simulink model "RflysimIndoorController_r2018b_N12_V9"  (R2018b)
settings: Solver=ode4  StartTime=0.0  StopTime=inf  FixedStep=ts  MaxStep=0.6  RelTol=1e-3
values from neighbouring files (symbols this model uses):
  l_v = 5    [RflyMain.m]    (also in RflyMain_N12_V6.m; RflyMain_N6_V3.m; RflyMain_N6_V4.m; RflyMain_V2.m)
  p_target = [200,10]    [RflyMain.m]    (also in RflyMain_N12_V6.m; RflyMain_N6_V3.m; RflyMain_N6_V4.m; RflyMain_V2.m)
  ra = 0.6    [RflyMain.m]    (also in RflyMain_N12_V6.m; RflyMain_N6_V3.m; RflyMain_N6_V4.m; RflyMain_V2.m)
  rs = 0.25    [RflyMain.m]    (also in RflyMain_N12_V6.m; RflyMain_N6_V3.m; RflyMain_N6_V4.m; RflyMain_V2.m)
  rt_a = 1.5    [RflyMain_N12_V6.m]
  rt_s = 0.25    [RflyMain_N12_V6.m]
  ts = [0 0]    [QuadModel2D.m]    (also in RflyMain.m = 0.01; RflyMain_N12_V6.m = 0.05; RflyMain_N6_V3.m = 0.05; RflyMain_N6_V4.m = 0.05)
  v_max = 2    [RflyMain.m]    (also in RflyMain_N12_V6.m = 3; RflyMain_N6_V3.m = 3; RflyMain_N6_V4.m = 3; RflyMain_V2.m = 3)
undefined symbols (not defined in the file or in its folder): Twist
libraries: robotlib x96, aerolibanimutils x1
(part 1 of 2)
settings Model: Creator=51078  LastModifiedBy=51078
settings OptimizationCC: EnhancedBackFolding=on  PassReuseOutputArgsAs=Individual arguments  ZeroExternalMemoryAtStartup=off  ZeroInternalMemoryAtStartup=off  MaxStackSize=64  OptimizeBlockOrder=speed  DifferentSizesBufferReuse=on  OptimizationCustomize=off
settings DebuggingCC: RTPrefix=warning  ParameterTunabilityLossMsg=error
settings HardwareCC: ProdBitPerPointer=32  ProdBitPerSizeT=32  ProdBitPerPtrDiffT=32  ProdLargestAtomicFloat=None  ProdIntDivRoundTo=Undefined  ProdEndianess=Unspecified  ProdWordSize=32  ProdHWDeviceType=Generic->Unspecified (assume 32-bit Generic)
settings SFSimCC: SimUseLocalCustomCode=off  MATLABDynamicMemAlloc=off
settings RTWCC: SystemTargetFile=ert.tlc  HardwareBoard=Robot Operating System (ROS)  TLCOptions="-aInlineSetEventsForThisBaseRateFcn=TLC_FALSE -aSuppressMultiTaskScheduler=TLC_FALSE  -aRateBasedStepFcn=0"  TemplateMakefile=ert_default_tmf  RTWUseLocalCustomCode=off  Toolchain=Catkin  TargetLang=C++
settings CodeAppCC: ForceParamTrailComments=on  IgnoreCustomStorageClasses=off  OperatorAnnotations=on  SimulinkDataObjDesc=on  SFDataObjDesc=on  InsertBlockDesc=on
settings ERTTargetCC: SupportVariableSizeSignals=on

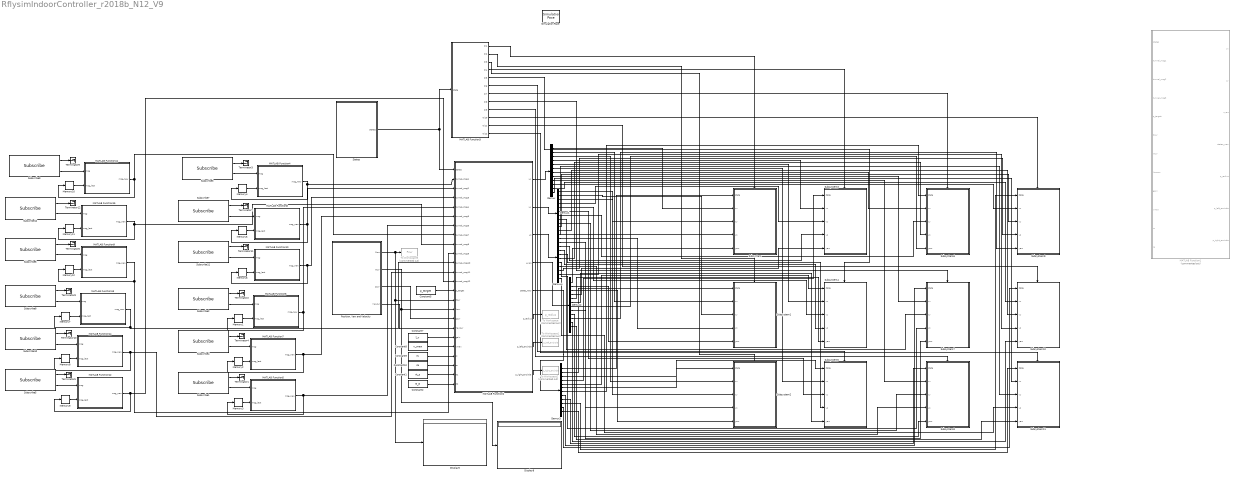
== system RflysimIndoorController_r2018b_N12_V9 ==
  Constant1 : Constant  Value=rt_s
  Constant10 : Constant  Value=ra
  Constant2 : Constant  Value=rt_a
  Constant5 : Constant  Value=p_target
  Constant7 : Constant  Value=l_v
  Constant8 : Constant  Value=v_max
  Constant9 : Constant  Value=rs
  Demux{,1..4} (5 alike) : Demux  Outputs=12
  Display6 : Display
  Display8 : Display
  MATLAB Function1 : MATLAB Function  Commented=on  TreatAsAtomicUnit=on
  MATLAB Function10 : MATLAB Function  TreatAsAtomicUnit=on
  MATLAB Function11 : MATLAB Function  TreatAsAtomicUnit=on
  MATLAB Function12 : MATLAB Function  TreatAsAtomicUnit=on
  MATLAB Function13 : MATLAB Function  TreatAsAtomicUnit=on
  MATLAB Function14 : MATLAB Function  TreatAsAtomicUnit=on
  MATLAB Function15 : MATLAB Function  TreatAsAtomicUnit=on
  MATLAB Function2 : MATLAB Function  TreatAsAtomicUnit=on
  MATLAB Function3 : MATLAB Function  TreatAsAtomicUnit=on
  MATLAB Function4 : MATLAB Function  TreatAsAtomicUnit=on
  MATLAB Function5 : MATLAB Function  TreatAsAtomicUnit=on
  MATLAB Function6 : MATLAB Function  TreatAsAtomicUnit=on
  MATLAB Function7 : MATLAB Function  TreatAsAtomicUnit=on
  MATLAB Function8 : MATLAB Function  TreatAsAtomicUnit=on
  MATLAB Function9 : MATLAB Function  TreatAsAtomicUnit=on
  Memory{1..12} (12 alike) : Memory
  "Position, Yaw and Velocity" : Subsystem
  Simulation Pace : aerolibanimutils/Simulation Pace  SimulationPace=1  SleepMode=MATLAB Thread  OutputPaceError=off  SampleTime=ts
  States : Subsystem
  Subscribe1 : robotlib/Subscribe  topicSource=Specify your own  topic=/drone_6/decision_info  messageType=swarm_msgs/Pipeline  sampleTime=-1  messageQueueLength=1
  Subscribe10 : robotlib/Subscribe  topicSource=Specify your own  topic=/drone_11/decision_info  messageType=swarm_msgs/Pipeline  sampleTime=-1  messageQueueLength=1
  Subscribe11 : robotlib/Subscribe  topicSource=Select from ROS network  topic=/drone_3/decision_info  messageType=swarm_msgs/Pipeline  sampleTime=-1  messageQueueLength=1
  Subscribe12 : robotlib/Subscribe  topicSource=Specify your own  topic=/drone_8/decision_info  messageType=swarm_msgs/Pipeline  sampleTime=-1  messageQueueLength=1
  Subscribe2 : robotlib/Subscribe  topicSource=Specify your own  topic=/drone_4/decision_info  messageType=swarm_msgs/Pipeline  sampleTime=-1  messageQueueLength=1
  Subscribe3 : robotlib/Subscribe  topicSource=Select from ROS network  topic=/drone_1/decision_info  messageType=swarm_msgs/Pipeline  sampleTime=-1  messageQueueLength=1
  Subscribe4 : robotlib/Subscribe  topicSource=Specify your own  topic=/drone_5/decision_info  messageType=swarm_msgs/Pipeline  sampleTime=-1  messageQueueLength=1
  Subscribe5 : robotlib/Subscribe  topicSource=Specify your own  topic=/drone_12/decision_info  messageType=swarm_msgs/Pipeline  sampleTime=-1  messageQueueLength=1
  Subscribe6 : robotlib/Subscribe  topicSource=Specify your own  topic=/drone_9/decision_info  messageType=swarm_msgs/Pipeline  sampleTime=-1  messageQueueLength=1
  Subscribe7 : robotlib/Subscribe  topicSource=Select from ROS network  topic=/drone_2/decision_info  messageType=swarm_msgs/Pipeline  sampleTime=-1  messageQueueLength=1
  Subscribe8 : robotlib/Subscribe  topicSource=Specify your own  topic=/drone_10/decision_info  messageType=swarm_msgs/Pipeline  sampleTime=-1  messageQueueLength=1
  Subscribe9 : robotlib/Subscribe  topicSource=Specify your own  topic=/drone_7/decision_info  messageType=swarm_msgs/Pipeline  sampleTime=-1  messageQueueLength=1
  Subsystem : Subsystem
  Subsystem1 : Subsystem
  Subsystem10 : Subsystem
  Subsystem11 : Subsystem
  Subsystem2 : Subsystem
  Subsystem3 : Subsystem
  Subsystem4 : Subsystem
  Subsystem5 : Subsystem
  Subsystem6 : Subsystem
  Subsystem7 : Subsystem
  Subsystem8 : Subsystem
  Subsystem9 : Subsystem
  Terminator{1..12} (12 alike) : Terminator
  To Workspace : ToWorkspace  Commented=on  VariableName=p_radius  SaveFormat=Timeseries  SampleTime=-1
  To Workspace1 : ToWorkspace  Commented=on  VariableName=p_left_encircle  SaveFormat=Timeseries  SampleTime=-1
  To Workspace2 : ToWorkspace  Commented=on  VariableName=p_right_encircle  SaveFormat=Timeseries  SampleTime=-1
  To Workspace3 : ToWorkspace  Commented=on  VariableName=Pcur  SaveFormat=Timeseries  SampleTime=-1
  wires:
  Constant9/1 -> MATLAB Function2/21(rs)
  MATLAB Function2/4(uyaw) -> Demux2/1
  Constant5/1 -> MATLAB Function2/14(p_target)
  Constant7/1 -> MATLAB Function2/19(gain)
  Constant10/1 -> MATLAB Function2/22(ra)
  MATLAB Function2/1(ux) -> Demux/1
  Constant8/1 -> MATLAB Function2/20(vmax)
  MATLAB Function2/5(states_new) -> Demux3/1
  MATLAB Function2/2(uy) -> Demux1/1
  Subscribe3/1 -> Terminator3/1
  MATLAB Function4/1(msg_new) -> Memory4/1, MATLAB Function2/2(tunnel_msg1)
  Subscribe3/2 -> MATLAB Function4/1(msg)
  Memory4/1 -> MATLAB Function4/2(msg_last)
  MATLAB Function2/6(p_radius) -> To Workspace/1
  MATLAB Function2/7(p_left_encircle) -> To Workspace1/1
  MATLAB Function2/8(p_right_encircle) -> To Workspace2/1
  Subscribe7/1 -> Terminator7/1
  Subscribe7/2 -> MATLAB Function8/1(msg)
  Memory5/1 -> MATLAB Function8/2(msg_last)
  MATLAB Function8/1(msg_new) -> MATLAB Function2/3(tunnel_msg2), Memory5/1
  Memory6/1 -> MATLAB Function10/2(msg_last)
  Subscribe11/1 -> Terminator11/1
  Subscribe11/2 -> MATLAB Function10/1(msg)
  MATLAB Function10/1(msg_new) -> Memory6/1, MATLAB Function2/4(tunnel_msg3)
  Demux/1 -> Subsystem/2(vx)
  Demux/2 -> Subsystem1/2(vx)
  Demux/3 -> Subsystem2/2(vx)
  Demux1/1 -> Subsystem/3(vy)
  Demux1/2 -> Subsystem1/3(vy)
  Demux1/3 -> Subsystem2/3(vy)
  Demux2/1 -> Subsystem/5(yaw)
  Demux2/2 -> Subsystem1/5(yaw)
  Demux2/3 -> Subsystem2/5(yaw)
  Demux3/1 -> Subsystem/1(state)
  Demux3/2 -> Subsystem1/1(state)
  Demux3/3 -> Subsystem2/1(state)
  MATLAB Function3/1(tri1) -> Subsystem/Enable
  MATLAB Function3/2(tri2) -> Subsystem1/Enable
  MATLAB Function3/3(tri3) -> Subsystem2/Enable
  States/1(States) -> MATLAB Function2/1(states), MATLAB Function3/1(state)
  "Position, Yaw and Velocity"/2(Vcur) -> Display8/1, MATLAB Function2/16(Vcur)
  "Position, Yaw and Velocity"/1(Pcur) -> Display6/1, MATLAB Function2/15(Pcur), To Workspace3/1
  "Position, Yaw and Velocity"/4(Yawcur) -> MATLAB Function2/18(Yawcur)
  "Position, Yaw and Velocity"/3(Zcur) -> MATLAB Function2/17(Zcur)
  MATLAB Function2/3(uz) -> Demux4/1
  Demux4/1 -> Subsystem/4(vz)
  Demux4/2 -> Subsystem1/4(vz)
  Demux4/3 -> Subsystem2/4(vz)
  Subscribe2/2 -> MATLAB Function6/1(msg)
  Subscribe1/1 -> Terminator1/1
  Subscribe2/1 -> Terminator2/1
  Subscribe4/1 -> Terminator4/1
  Subscribe4/2 -> MATLAB Function7/1(msg)
  Subscribe1/2 -> MATLAB Function5/1(msg)
  Memory1/1 -> MATLAB Function6/2(msg_last)
  MATLAB Function6/1(msg_new) -> Memory1/1, MATLAB Function2/5(tunnel_msg4)
  MATLAB Function5/1(msg_new) -> MATLAB Function2/7(tunnel_msg6), Memory3/1
  MATLAB Function7/1(msg_new) -> MATLAB Function2/6(tunnel_msg5), Memory2/1
  Memory3/1 -> MATLAB Function5/2(msg_last)
  Memory2/1 -> MATLAB Function7/2(msg_last)
  MATLAB Function3/4(tri4) -> Subsystem3/Enable
  MATLAB Function3/5(tri5) -> Subsystem4/Enable
  MATLAB Function3/6(tri6) -> Subsystem5/Enable
  Demux/4 -> Subsystem3/2(vx)
  Demux/5 -> Subsystem4/2(vx)
  Demux/6 -> Subsystem5/2(vx)
  Demux1/4 -> Subsystem3/3(vy)
  Demux1/5 -> Subsystem4/3(vy)
  Demux1/6 -> Subsystem5/3(vy)
  Demux4/4 -> Subsystem3/4(vz)
  Demux4/5 -> Subsystem4/4(vz)
  Demux4/6 -> Subsystem5/4(vz)
  Demux2/4 -> Subsystem3/5(yaw)
  Demux2/5 -> Subsystem4/5(yaw)
  Demux2/6 -> Subsystem5/5(yaw)
  Demux3/4 -> Subsystem3/1(state)
  Demux3/5 -> Subsystem4/1(state)
  Demux3/6 -> Subsystem5/1(state)
  Constant1/1 -> MATLAB Function2/23(rt1)
  Constant2/1 -> MATLAB Function2/24(rt2)
  Subscribe8/1 -> Terminator8/1
  Subscribe9/2 -> MATLAB Function11/1(msg)
  Subscribe6/1 -> Terminator6/1
  Memory7/1 -> MATLAB Function13/2(msg_last)
  MATLAB Function12/1(msg_new) -> MATLAB Function2/13(tunnel_msg12), Memory9/1
  Subscribe5/1 -> Terminator5/1
  Memory11/1 -> MATLAB Function15/2(msg_last)
  Subscribe6/2 -> MATLAB Function9/1(msg)
  Memory8/1 -> MATLAB Function14/2(msg_last)
  MATLAB Function14/1(msg_new) -> MATLAB Function2/12(tunnel_msg11), Memory8/1
  MATLAB Function13/1(msg_new) -> MATLAB Function2/11(tunnel_msg10), Memory7/1
  Memory12/1 -> MATLAB Function9/2(msg_last)
  Memory10/1 -> MATLAB Function11/2(msg_last)
  Subscribe10/2 -> MATLAB Function14/1(msg)
  Subscribe5/2 -> MATLAB Function12/1(msg)
  Subscribe12/2 -> MATLAB Function15/1(msg)
  Memory9/1 -> MATLAB Function12/2(msg_last)
  MATLAB Function15/1(msg_new) -> MATLAB Function2/9(tunnel_msg8), Memory11/1
  Subscribe9/1 -> Terminator9/1
  MATLAB Function11/1(msg_new) -> MATLAB Function2/8(tunnel_msg7), Memory10/1
  MATLAB Function9/1(msg_new) -> MATLAB Function2/10(tunnel_msg9), Memory12/1
  Subscribe8/2 -> MATLAB Function13/1(msg)
  Subscribe12/1 -> Terminator12/1
  Subscribe10/1 -> Terminator10/1
  MATLAB Function3/7(tri7) -> Subsystem6/Enable
  MATLAB Function3/8(tri8) -> Subsystem7/Enable
  MATLAB Function3/9(tri9) -> Subsystem8/Enable
  MATLAB Function3/10(tri10) -> Subsystem9/Enable
  MATLAB Function3/11(tri11) -> Subsystem10/Enable
  MATLAB Function3/12(tri12) -> Subsystem11/Enable
  Demux/7 -> Subsystem6/2(vx)
  Demux/8 -> Subsystem7/2(vx)
  Demux/9 -> Subsystem8/2(vx)
  Demux/10 -> Subsystem9/2(vx)
  Demux/11 -> Subsystem10/2(vx)
  Demux/12 -> Subsystem11/2(vx)
  Demux1/7 -> Subsystem6/3(vy)
  Demux1/8 -> Subsystem7/3(vy)
  Demux1/9 -> Subsystem8/3(vy)
  Demux1/10 -> Subsystem9/3(vy)
  Demux1/11 -> Subsystem10/3(vy)
  Demux1/12 -> Subsystem11/3(vy)
  Demux4/7 -> Subsystem6/4(vz)
  Demux4/8 -> Subsystem7/4(vz)
  Demux4/9 -> Subsystem8/4(vz)
  Demux4/10 -> Subsystem9/4(vz)
  Demux4/11 -> Subsystem10/4(vz)
  Demux4/12 -> Subsystem11/4(vz)
  Demux2/7 -> Subsystem6/5(yaw)
  Demux2/8 -> Subsystem7/5(yaw)
  Demux2/9 -> Subsystem8/5(yaw)
  Demux2/10 -> Subsystem9/5(yaw)
  Demux2/11 -> Subsystem10/5(yaw)
  Demux2/12 -> Subsystem11/5(yaw)
  Demux3/7 -> Subsystem6/1(state)
  Demux3/8 -> Subsystem7/1(state)
  Demux3/9 -> Subsystem8/1(state)
  Demux3/10 -> Subsystem9/1(state)
  Demux3/11 -> Subsystem10/1(state)
  Demux3/12 -> Subsystem11/1(state)

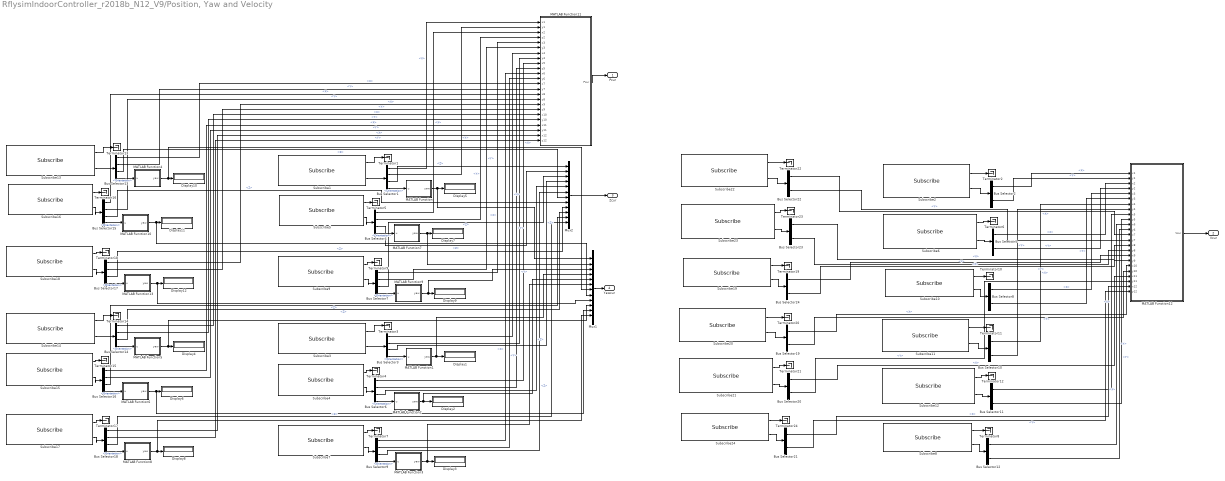
== system RflysimIndoorController_r2018b_N12_V9/Position, Yaw and Velocity ==
  Bus Selector{1,3..4,6..7,9,13..18} (12 alike) : BusSelector  OutputSignals=Pose.Position.X,Pose.Position.Y,Pose.Position.Z,Pose.Orientation
  Bus Selector{2,5,8,10..12,19..24} (12 alike) : BusSelector  OutputSignals=Twist.Linear.X,Twist.Linear.Y
  Display{1..12} (12 alike) : Display
  MATLAB Function : MATLAB Function  TreatAsAtomicUnit=on
  MATLAB Function1 : MATLAB Function  TreatAsAtomicUnit=on
  MATLAB Function10 : MATLAB Function  TreatAsAtomicUnit=on
  MATLAB Function11 : MATLAB Function  TreatAsAtomicUnit=on
  MATLAB Function12 : MATLAB Function  TreatAsAtomicUnit=on
  MATLAB Function13 : MATLAB Function  TreatAsAtomicUnit=on
  MATLAB Function2 : MATLAB Function  TreatAsAtomicUnit=on
  MATLAB Function3 : MATLAB Function  TreatAsAtomicUnit=on
  MATLAB Function4 : MATLAB Function  TreatAsAtomicUnit=on
  MATLAB Function5 : MATLAB Function  TreatAsAtomicUnit=on
  MATLAB Function6 : MATLAB Function  TreatAsAtomicUnit=on
  MATLAB Function7 : MATLAB Function  TreatAsAtomicUnit=on
  MATLAB Function8 : MATLAB Function  TreatAsAtomicUnit=on
  MATLAB Function9 : MATLAB Function  TreatAsAtomicUnit=on
  Mux1 : Mux  Inputs=12
  Mux2 : Mux  Inputs=12
  Subscribe1 : robotlib/Subscribe  topicSource=Select from ROS network  topic=/drone_1/mavros/local_position/pose_cor  messageType=geometry_msgs/PoseStamped  sampleTime=-1  messageQueueLength=1
  Subscribe10 : robotlib/Subscribe  topicSource=Select from ROS network  topic=/drone_3/mavros/local_position/velocity_local  messageType=geometry_msgs/TwistStamped  sampleTime=-1  messageQueueLength=1
  Subscribe11 : robotlib/Subscribe  topicSource=Specify your own  topic=/drone_4/mavros/local_position/velocity_local  messageType=geometry_msgs/TwistStamped  sampleTime=-1  messageQueueLength=1
  Subscribe12 : robotlib/Subscribe  topicSource=Specify your own  topic=/drone_5/mavros/local_position/velocity_local  messageType=geometry_msgs/TwistStamped  sampleTime=-1  messageQueueLength=1
  Subscribe13 : robotlib/Subscribe  topicSource=Specify your own  topic=/drone_7/mavros/local_position/pose_cor  messageType=geometry_msgs/PoseStamped  sampleTime=-1  messageQueueLength=1
  Subscribe14 : robotlib/Subscribe  topicSource=Specify your own  topic=/drone_10/mavros/local_position/pose_cor  messageType=geometry_msgs/PoseStamped  sampleTime=-1  messageQueueLength=1
  Subscribe15 : robotlib/Subscribe  topicSource=Specify your own  topic=/drone_11/mavros/local_position/pose_cor  messageType=geometry_msgs/PoseStamped  sampleTime=-1  messageQueueLength=1
  Subscribe16 : robotlib/Subscribe  topicSource=Specify your own  topic=/drone_8/mavros/local_position/pose_cor  messageType=geometry_msgs/PoseStamped  sampleTime=-1  messageQueueLength=1
  Subscribe17 : robotlib/Subscribe  topicSource=Specify your own  topic=/drone_12/mavros/local_position/pose_cor  messageType=geometry_msgs/PoseStamped  sampleTime=-1  messageQueueLength=1
  Subscribe18 : robotlib/Subscribe  topicSource=Specify your own  topic=/drone_9/mavros/local_position/pose_cor  messageType=geometry_msgs/PoseStamped  sampleTime=-1  messageQueueLength=1
  Subscribe19 : robotlib/Subscribe  topicSource=Specify your own  topic=/drone_9/mavros/local_position/velocity_local  messageType=geometry_msgs/TwistStamped  sampleTime=-1  messageQueueLength=1
  Subscribe2 : robotlib/Subscribe  topicSource=Select from ROS network  topic=/drone_1/mavros/local_position/velocity_local  messageType=geometry_msgs/TwistStamped  sampleTime=-1  messageQueueLength=1
  Subscribe20 : robotlib/Subscribe  topicSource=Specify your own  topic=/drone_10/mavros/local_position/velocity_local  messageType=geometry_msgs/TwistStamped  sampleTime=-1  messageQueueLength=1
  Subscribe21 : robotlib/Subscribe  topicSource=Specify your own  topic=/drone_11/mavros/local_position/velocity_local  messageType=geometry_msgs/TwistStamped  sampleTime=-1  messageQueueLength=1
  Subscribe22 : robotlib/Subscribe  topicSource=Specify your own  topic=/drone_7/mavros/local_position/velocity_local  messageType=geometry_msgs/TwistStamped  sampleTime=-1  messageQueueLength=1
  Subscribe23 : robotlib/Subscribe  topicSource=Specify your own  topic=/drone_8/mavros/local_position/velocity_local  messageType=geometry_msgs/TwistStamped  sampleTime=-1  messageQueueLength=1
  Subscribe24 : robotlib/Subscribe  topicSource=Specify your own  topic=/drone_12/mavros/local_position/velocity_local  messageType=geometry_msgs/TwistStamped  sampleTime=-1  messageQueueLength=1
  Subscribe3 : robotlib/Subscribe  topicSource=Specify your own  topic=/drone_4/mavros/local_position/pose_cor  messageType=geometry_msgs/PoseStamped  sampleTime=-1  messageQueueLength=1
  Subscribe4 : robotlib/Subscribe  topicSource=Specify your own  topic=/drone_5/mavros/local_position/pose_cor  messageType=geometry_msgs/PoseStamped  sampleTime=-1  messageQueueLength=1
  Subscribe5 : robotlib/Subscribe  topicSource=Select from ROS network  topic=/drone_2/mavros/local_position/pose_cor  messageType=geometry_msgs/PoseStamped  sampleTime=-1  messageQueueLength=1
  Subscribe6 : robotlib/Subscribe  topicSource=Select from ROS network  topic=/drone_2/mavros/local_position/velocity_local  messageType=geometry_msgs/TwistStamped  sampleTime=-1  messageQueueLength=1
  Subscribe7 : robotlib/Subscribe  topicSource=Specify your own  topic=/drone_6/mavros/local_position/pose_cor  messageType=geometry_msgs/PoseStamped  sampleTime=-1  messageQueueLength=1
  Subscribe8 : robotlib/Subscribe  topicSource=Specify your own  topic=/drone_6/mavros/local_position/velocity_local  messageType=geometry_msgs/TwistStamped  sampleTime=-1  messageQueueLength=1
  Subscribe9 : robotlib/Subscribe  topicSource=Select from ROS network  topic=/drone_3/mavros/local_position/pose_cor  messageType=geometry_msgs/PoseStamped  sampleTime=-1  messageQueueLength=1
  Terminator{1..24} (24 alike) : Terminator
  Pcur : Outport
  Vcur : Outport  Port=2
  Zcur : Outport  Port=3
  Yawcur : Outport  Port=4
  wires:
  Subscribe1/1 -> Terminator1/1
  Mux1/1 -> Yawcur/1
  Subscribe10/1 -> Terminator10/1
  MATLAB Function/1(yaw) -> Mux1/1, Display5/1
  Subscribe9/2 -> Bus Selector7/1
  Bus Selector7/3 -> Mux2/3  "<Z>"
  Bus Selector4/3 -> Mux2/2  "<Z>"
  Subscribe5/1 -> Terminator5/1
  Subscribe6/2 -> Bus Selector5/1
  Subscribe9/1 -> Terminator9/1
  Subscribe10/2 -> Bus Selector8/1
  Bus Selector2/2 -> MATLAB Function12/2(y1)  "<Y>"
  Bus Selector4/1 -> MATLAB Function11/3(x2)  "<X>"
  Bus Selector1/1 -> MATLAB Function11/1(x1)  "<X>"
  Subscribe2/1 -> Terminator2/1
  Subscribe2/2 -> Bus Selector2/1
  Bus Selector5/2 -> MATLAB Function12/4(y2)  "<Y>"
  MATLAB Function12/1(Vcur) -> Vcur/1
  Bus Selector8/1 -> MATLAB Function12/5(x3)  "<X>"
  Bus Selector5/1 -> MATLAB Function12/3(x2)  "<X>"
  Subscribe1/2 -> Bus Selector1/1
  Bus Selector7/2 -> MATLAB Function11/6(y3)  "<Y>"
  Bus Selector8/2 -> MATLAB Function12/6(y3)  "<Y>"
  Bus Selector4/2 -> MATLAB Function11/4(y2)  "<Y>"
  Subscribe6/1 -> Terminator6/1
  Bus Selector7/1 -> MATLAB Function11/5(x3)  "<X>"
  Bus Selector4/4 -> MATLAB Function7/1(u)  "<Orientation>"
  Bus Selector1/4 -> MATLAB Function/1(u)  "<Orientation>"
  MATLAB Function11/1(Pcur) -> Pcur/1
  Bus Selector7/4 -> MATLAB Function9/1(u)  "<Orientation>"
  MATLAB Function7/1(yaw) -> Mux1/2, Display7/1
  Mux2/1 -> Zcur/1
  Bus Selector2/1 -> MATLAB Function12/1(x1)  "<X>"
  MATLAB Function9/1(yaw) -> Mux1/3, Display9/1
  Bus Selector1/2 -> MATLAB Function11/2(y1)  "<Y>"
  Subscribe5/2 -> Bus Selector4/1
  Bus Selector1/3 -> Mux2/1  "<Z>"
  Subscribe4/1 -> Terminator4/1
  Bus Selector3/4 -> MATLAB Function1/1(u)  "<Orientation>"
  Bus Selector9/4 -> MATLAB Function3/1(u)  "<Orientation>"
  Subscribe7/1 -> Terminator7/1
  MATLAB Function3/1(yaw) -> Mux1/6, Display3/1
  Subscribe3/1 -> Terminator3/1
  MATLAB Function2/1(yaw) -> Mux1/5, Display2/1
  Bus Selector6/4 -> MATLAB Function2/1(u)  "<Orientation>"
  MATLAB Function1/1(yaw) -> Mux1/4, Display1/1
  Subscribe7/2 -> Bus Selector9/1
  Subscribe4/2 -> Bus Selector6/1
  Subscribe3/2 -> Bus Selector3/1
  Bus Selector3/1 -> MATLAB Function11/7(x4)  "<X>"
  Bus Selector3/2 -> MATLAB Function11/8(y4)  "<Y>"
  Bus Selector6/1 -> MATLAB Function11/9(x5)  "<X>"
  Bus Selector6/2 -> MATLAB Function11/10(y5)  "<Y>"
  Bus Selector9/1 -> MATLAB Function11/11(x6)  "<X>"
  Bus Selector9/2 -> MATLAB Function11/12(y6)  "<Y>"
  Bus Selector3/3 -> Mux2/4  "<Z>"
  Bus Selector6/3 -> Mux2/5  "<Z>"
  Bus Selector9/3 -> Mux2/6  "<Z>"
  Subscribe12/1 -> Terminator12/1
  Subscribe8/2 -> Bus Selector12/1
  Subscribe12/2 -> Bus Selector11/1
  Subscribe11/2 -> Bus Selector10/1
  Subscribe11/1 -> Terminator11/1
  Subscribe8/1 -> Terminator8/1
  Bus Selector10/1 -> MATLAB Function12/7(x4)  "<X>"
  Bus Selector10/2 -> MATLAB Function12/8(y4)  "<Y>"
  Bus Selector11/1 -> MATLAB Function12/9(x5)  "<X>"
  Bus Selector11/2 -> MATLAB Function12/10(y5)  "<Y>"
  Bus Selector12/1 -> MATLAB Function12/11(x6)  "<X>"
  Bus Selector12/2 -> MATLAB Function12/12(y6)  "<Y>"
  Subscribe13/2 -> Bus Selector13/1
  MATLAB Function4/1(yaw) -> Mux1/7, Display10/1
  Bus Selector13/4 -> MATLAB Function4/1(u)  "<Orientation>"
  MATLAB Function13/1(yaw) -> Mux1/9, Display12/1
  Subscribe16/1 -> Terminator16/1
  Bus Selector14/4 -> MATLAB Function5/1(u)  "<Orientation>"
  Subscribe14/1 -> Terminator14/1
  MATLAB Function10/1(yaw) -> Mux1/8, Display11/1
  MATLAB Function6/1(yaw) -> Mux1/11, Display6/1
  MATLAB Function5/1(yaw) -> Mux1/10, Display4/1
  Subscribe17/1 -> Terminator17/1
  Subscribe15/2 -> Bus Selector16/1
  Subscribe15/1 -> Terminator15/1
  Bus Selector18/4 -> MATLAB Function8/1(u)  "<Orientation>"
  MATLAB Function8/1(yaw) -> Mux1/12, Display8/1
  Subscribe14/2 -> Bus Selector14/1
  Subscribe13/1 -> Terminator13/1
  Bus Selector15/4 -> MATLAB Function10/1(u)  "<Orientation>"
  Bus Selector17/4 -> MATLAB Function13/1(u)  "<Orientation>"
  Subscribe18/2 -> Bus Selector17/1
  Bus Selector16/4 -> MATLAB Function6/1(u)  "<Orientation>"
  Subscribe18/1 -> Terminator18/1
  Subscribe17/2 -> Bus Selector18/1
  Subscribe16/2 -> Bus Selector15/1
  Bus Selector13/1 -> MATLAB Function11/13(x7)  "<X>"
  Bus Selector13/2 -> MATLAB Function11/14(y7)  "<Y>"
  Bus Selector15/1 -> MATLAB Function11/15(x8)  "<X>"
  Bus Selector15/2 -> MATLAB Function11/16(y8)  "<Y>"
  Bus Selector17/1 -> MATLAB Function11/17(x9)  "<X>"
  Bus Selector17/2 -> MATLAB Function11/18(y9)  "<Y>"
  Bus Selector14/1 -> MATLAB Function11/19(x10)  "<X>"
  Bus Selector14/2 -> MATLAB Function11/20(y10)  "<Y>"
  Bus Selector16/1 -> MATLAB Function11/21(x11)  "<X>"
  Bus Selector16/2 -> MATLAB Function11/22(y11)  "<Y>"
  Bus Selector18/1 -> MATLAB Function11/23(x12)  "<X>"
  Bus Selector18/2 -> MATLAB Function11/24(y12)  "<Y>"
  Bus Selector13/3 -> Mux2/7  "<Z>"
  Bus Selector15/3 -> Mux2/8  "<Z>"
  Bus Selector17/3 -> Mux2/9  "<Z>"
  Bus Selector14/3 -> Mux2/10  "<Z>"
  Bus Selector16/3 -> Mux2/11  "<Z>"
  Bus Selector18/3 -> Mux2/12  "<Z>"
  Subscribe23/1 -> Terminator23/1
  Subscribe24/1 -> Terminator24/1
  Subscribe23/2 -> Bus Selector23/1
  Subscribe20/2 -> Bus Selector19/1
  Subscribe24/2 -> Bus Selector21/1
  Subscribe21/2 -> Bus Selector20/1
  Subscribe22/2 -> Bus Selector22/1
  Subscribe21/1 -> Terminator21/1
  Subscribe20/1 -> Terminator20/1
  Subscribe19/1 -> Terminator19/1
  Subscribe19/2 -> Bus Selector24/1
  Subscribe22/1 -> Terminator22/1
  Bus Selector22/1 -> MATLAB Function12/13(x7)  "<X>"
  Bus Selector22/2 -> MATLAB Function12/14(y7)  "<Y>"
  Bus Selector23/1 -> MATLAB Function12/15(x8)  "<X>"
  Bus Selector23/2 -> MATLAB Function12/16(y8)  "<Y>"
  Bus Selector24/1 -> MATLAB Function12/17(x9)  "<X>"
  Bus Selector24/2 -> MATLAB Function12/18(y9)  "<Y>"
  Bus Selector19/1 -> MATLAB Function12/19(x10)  "<X>"
  Bus Selector19/2 -> MATLAB Function12/20(y10)  "<Y>"
  Bus Selector20/1 -> MATLAB Function12/21(x11)  "<X>"
  Bus Selector20/2 -> MATLAB Function12/22(y11)  "<Y>"
  Bus Selector21/1 -> MATLAB Function12/23(x12)  "<X>"
  Bus Selector21/2 -> MATLAB Function12/24(y12)  "<Y>"

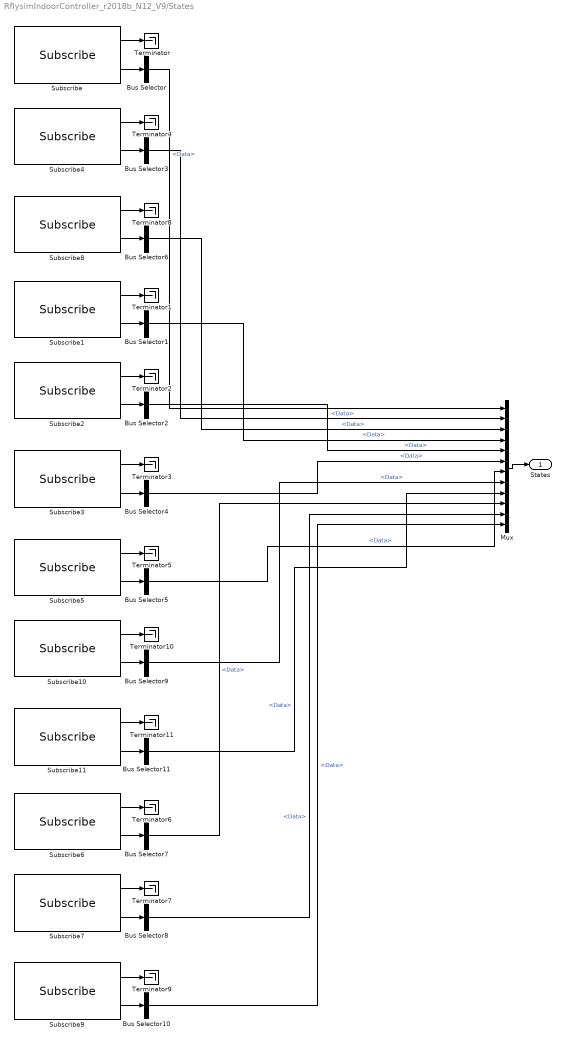
== system RflysimIndoorController_r2018b_N12_V9/States ==
  Bus Selector{,1..11} (12 alike) : BusSelector  OutputSignals=Data
  Mux : Mux  Inputs=12
  Subscribe : robotlib/Subscribe  topicSource=Select from ROS network  topic=/drone_1/state  messageType=std_msgs/UInt64  sampleTime=-1  messageQueueLength=1
  Subscribe1 : robotlib/Subscribe  topicSource=Specify your own  topic=/drone_4/state  messageType=std_msgs/UInt64  sampleTime=-1  messageQueueLength=1
  Subscribe10 : robotlib/Subscribe  topicSource=Specify your own  topic=/drone_8/state  messageType=std_msgs/UInt64  sampleTime=-1  messageQueueLength=1
  Subscribe11 : robotlib/Subscribe  topicSource=Specify your own  topic=/drone_9/state  messageType=std_msgs/UInt64  sampleTime=-1  messageQueueLength=1
  Subscribe2 : robotlib/Subscribe  topicSource=Specify your own  topic=/drone_5/state  messageType=std_msgs/UInt64  sampleTime=-1  messageQueueLength=1
  Subscribe3 : robotlib/Subscribe  topicSource=Specify your own  topic=/drone_6/state  messageType=std_msgs/UInt64  sampleTime=-1  messageQueueLength=1
  Subscribe4 : robotlib/Subscribe  topicSource=Select from ROS network  topic=/drone_2/state  messageType=std_msgs/UInt64  sampleTime=-1  messageQueueLength=1
  Subscribe5 : robotlib/Subscribe  topicSource=Specify your own  topic=/drone_7/state  messageType=std_msgs/UInt64  sampleTime=-1  messageQueueLength=1
  Subscribe6 : robotlib/Subscribe  topicSource=Specify your own  topic=/drone_10/state  messageType=std_msgs/UInt64  sampleTime=-1  messageQueueLength=1
  Subscribe7 : robotlib/Subscribe  topicSource=Specify your own  topic=/drone_11/state  messageType=std_msgs/UInt64  sampleTime=-1  messageQueueLength=1
  Subscribe8 : robotlib/Subscribe  topicSource=Select from ROS network  topic=/drone_3/state  messageType=std_msgs/UInt64  sampleTime=-1  messageQueueLength=1
  Subscribe9 : robotlib/Subscribe  topicSource=Specify your own  topic=/drone_12/state  messageType=std_msgs/UInt64  sampleTime=-1  messageQueueLength=1
  Terminator{,1..11} (12 alike) : Terminator
  States : Outport
  wires:
  Bus Selector3/1 -> Mux/2  "<Data>"
  Subscribe4/2 -> Bus Selector3/1
  Subscribe/2 -> Bus Selector/1
  Subscribe4/1 -> Terminator4/1
  Bus Selector6/1 -> Mux/3  "<Data>"
  Subscribe8/2 -> Bus Selector6/1
  Bus Selector/1 -> Mux/1  "<Data>"
  Subscribe/1 -> Terminator/1
  Subscribe8/1 -> Terminator8/1
  Mux/1 -> States/1
  Subscribe3/1 -> Terminator3/1
  Subscribe3/2 -> Bus Selector4/1
  Bus Selector4/1 -> Mux/6  "<Data>"
  Subscribe1/1 -> Terminator1/1
  Bus Selector1/1 -> Mux/4  "<Data>"
  Bus Selector2/1 -> Mux/5  "<Data>"
  Subscribe1/2 -> Bus Selector1/1
  Subscribe2/1 -> Terminator2/1
  Subscribe2/2 -> Bus Selector2/1
  Subscribe6/2 -> Bus Selector7/1
  Bus Selector8/1 -> Mux/11  "<Data>"
  Subscribe7/2 -> Bus Selector8/1
  Bus Selector11/1 -> Mux/9  "<Data>"
  Subscribe7/1 -> Terminator7/1
  Subscribe10/1 -> Terminator10/1
  Subscribe9/1 -> Terminator9/1
  Bus Selector7/1 -> Mux/10  "<Data>"
  Subscribe5/1 -> Terminator5/1
  Subscribe11/1 -> Terminator11/1
  Bus Selector5/1 -> Mux/7  "<Data>"
  Bus Selector9/1 -> Mux/8  "<Data>"
  Subscribe9/2 -> Bus Selector10/1
  Subscribe5/2 -> Bus Selector5/1
  Subscribe6/1 -> Terminator6/1
  Subscribe11/2 -> Bus Selector11/1
  Bus Selector10/1 -> Mux/12  "<Data>"
  Subscribe10/2 -> Bus Selector9/1

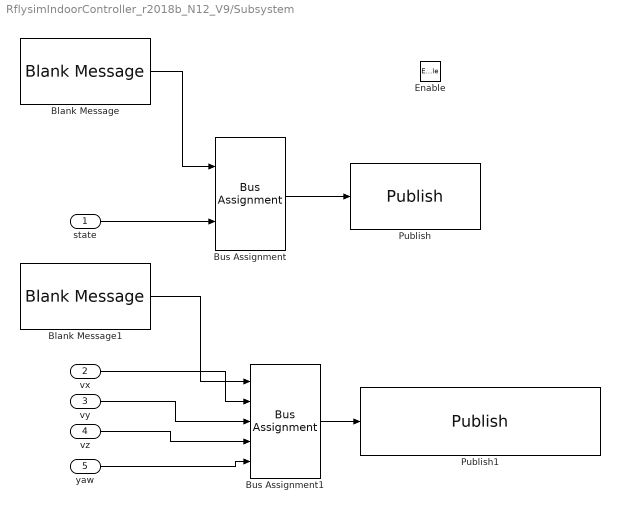
== system RflysimIndoorController_r2018b_N12_V9/Subsystem ==
  state : Inport
  vx : Inport  Port=2
  vy : Inport  Port=3
  vz : Inport  Port=4
  yaw : Inport  Port=5
  Enable : EnablePort
  Blank Message : robotlib/Blank Message  messageClass=Message  entityType=std_msgs/UInt64  messageType=std_msgs/UInt64  SampleTime=inf
  Blank Message1 : robotlib/Blank Message  messageClass=Message  entityType=geometry_msgs/TwistStamped  messageType=geometry_msgs/TwistStamped  SampleTime=inf
  Bus Assignment : BusAssignment  AssignedSignals=Data
  Bus Assignment1 : BusAssignment  AssignedSignals=Twist.Linear.X,Twist.Linear.Y,Twist.Linear.Z,Twist.Angular.Z
  Publish : robotlib/Publish  topicSource=Select from ROS network  topic=/drone_1/state  messageType=std_msgs/UInt64  messageQueueLength=1
  Publish1 : robotlib/Publish  topicSource=Select from ROS network  topic=/drone_1/mavros/setpoint_velocity/cmd_vel  messageType=geometry_msgs/TwistStamped  messageQueueLength=1
  wires:
  Blank Message/1 -> Bus Assignment/1
  state/1 -> Bus Assignment/2
  Bus Assignment/1 -> Publish/1
  Bus Assignment1/1 -> Publish1/1
  Blank Message1/1 -> Bus Assignment1/1
  vx/1 -> Bus Assignment1/2
  vy/1 -> Bus Assignment1/3
  yaw/1 -> Bus Assignment1/5
  vz/1 -> Bus Assignment1/4

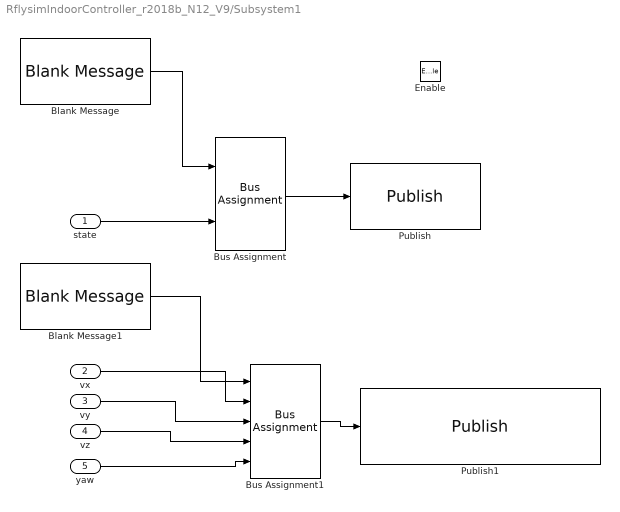
== system RflysimIndoorController_r2018b_N12_V9/Subsystem1 ==
  state : Inport
  vx : Inport  Port=2
  vy : Inport  Port=3
  vz : Inport  Port=4
  yaw : Inport  Port=5
  Enable : EnablePort
  Blank Message : robotlib/Blank Message  messageClass=Message  entityType=std_msgs/UInt64  messageType=std_msgs/UInt64  SampleTime=inf
  Blank Message1 : robotlib/Blank Message  messageClass=Message  entityType=geometry_msgs/TwistStamped  messageType=geometry_msgs/TwistStamped  SampleTime=inf
  Bus Assignment : BusAssignment  AssignedSignals=Data
  Bus Assignment1 : BusAssignment  AssignedSignals=Twist.Linear.X,Twist.Linear.Y,Twist.Linear.Z,Twist.Angular.Z
  Publish : robotlib/Publish  topicSource=Select from ROS network  topic=/drone_2/state  messageType=std_msgs/UInt64  messageQueueLength=1
  Publish1 : robotlib/Publish  topicSource=Select from ROS network  topic=/drone_2/mavros/setpoint_velocity/cmd_vel  messageType=geometry_msgs/TwistStamped  messageQueueLength=1
  wires:
  Blank Message/1 -> Bus Assignment/1
  state/1 -> Bus Assignment/2
  Bus Assignment/1 -> Publish/1
  Bus Assignment1/1 -> Publish1/1
  Blank Message1/1 -> Bus Assignment1/1
  vx/1 -> Bus Assignment1/2
  vy/1 -> Bus Assignment1/3
  yaw/1 -> Bus Assignment1/5
  vz/1 -> Bus Assignment1/4

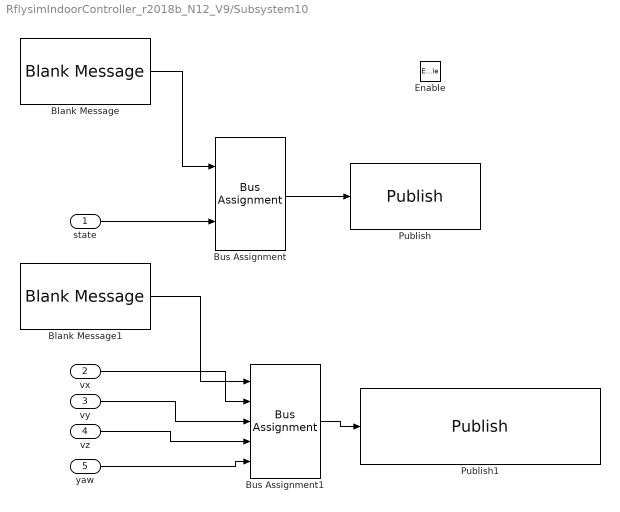
== system RflysimIndoorController_r2018b_N12_V9/Subsystem10 ==
  state : Inport
  vx : Inport  Port=2
  vy : Inport  Port=3
  vz : Inport  Port=4
  yaw : Inport  Port=5
  Enable : EnablePort
  Blank Message : robotlib/Blank Message  messageClass=Message  entityType=std_msgs/UInt64  messageType=std_msgs/UInt64  SampleTime=inf
  Blank Message1 : robotlib/Blank Message  messageClass=Message  entityType=geometry_msgs/TwistStamped  messageType=geometry_msgs/TwistStamped  SampleTime=inf
  Bus Assignment : BusAssignment  AssignedSignals=Data
  Bus Assignment1 : BusAssignment  AssignedSignals=Twist.Linear.X,Twist.Linear.Y,Twist.Linear.Z,Twist.Angular.Z
  Publish : robotlib/Publish  topicSource=Specify your own  topic=/drone_11/state  messageType=std_msgs/UInt64  messageQueueLength=1
  Publish1 : robotlib/Publish  topicSource=Specify your own  topic=/drone_11/mavros/setpoint_velocity/cmd_vel  messageType=geometry_msgs/TwistStamped  messageQueueLength=1
  wires:
  Blank Message/1 -> Bus Assignment/1
  state/1 -> Bus Assignment/2
  Bus Assignment/1 -> Publish/1
  Bus Assignment1/1 -> Publish1/1
  Blank Message1/1 -> Bus Assignment1/1
  vx/1 -> Bus Assignment1/2
  vy/1 -> Bus Assignment1/3
  yaw/1 -> Bus Assignment1/5
  vz/1 -> Bus Assignment1/4

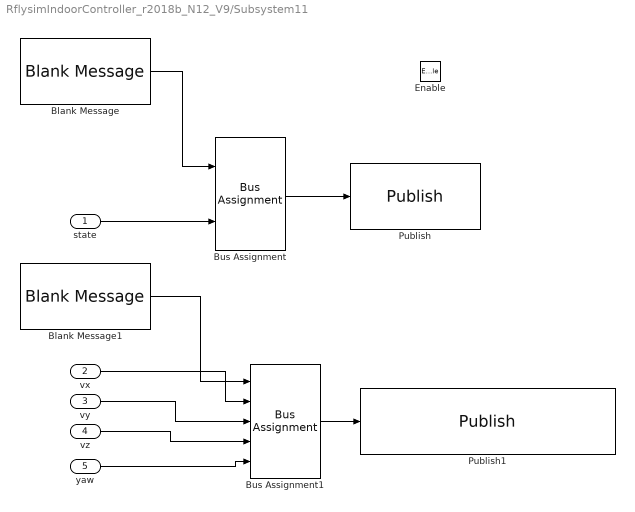
== system RflysimIndoorController_r2018b_N12_V9/Subsystem11 ==
  state : Inport
  vx : Inport  Port=2
  vy : Inport  Port=3
  vz : Inport  Port=4
  yaw : Inport  Port=5
  Enable : EnablePort
  Blank Message : robotlib/Blank Message  messageClass=Message  entityType=std_msgs/UInt64  messageType=std_msgs/UInt64  SampleTime=inf
  Blank Message1 : robotlib/Blank Message  messageClass=Message  entityType=geometry_msgs/TwistStamped  messageType=geometry_msgs/TwistStamped  SampleTime=inf
  Bus Assignment : BusAssignment  AssignedSignals=Data
  Bus Assignment1 : BusAssignment  AssignedSignals=Twist.Linear.X,Twist.Linear.Y,Twist.Linear.Z,Twist.Angular.Z
  Publish : robotlib/Publish  topicSource=Specify your own  topic=/drone_12/state  messageType=std_msgs/UInt64  messageQueueLength=1
  Publish1 : robotlib/Publish  topicSource=Specify your own  topic=/drone_12/mavros/setpoint_velocity/cmd_vel  messageType=geometry_msgs/TwistStamped  messageQueueLength=1
  wires:
  Blank Message/1 -> Bus Assignment/1
  state/1 -> Bus Assignment/2
  Bus Assignment/1 -> Publish/1
  Bus Assignment1/1 -> Publish1/1
  Blank Message1/1 -> Bus Assignment1/1
  vx/1 -> Bus Assignment1/2
  vy/1 -> Bus Assignment1/3
  yaw/1 -> Bus Assignment1/5
  vz/1 -> Bus Assignment1/4

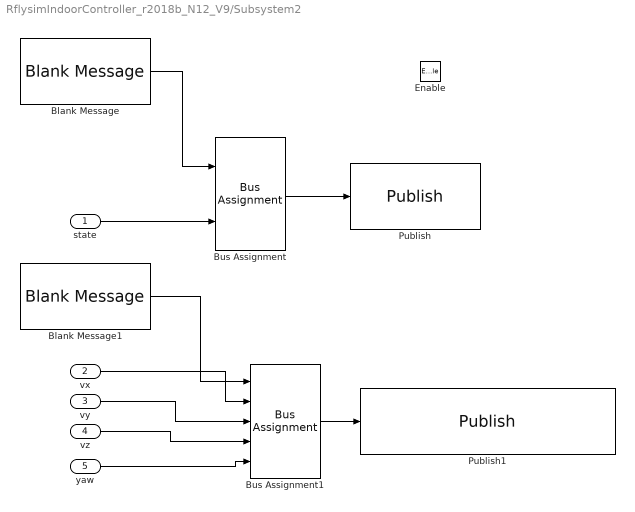
== system RflysimIndoorController_r2018b_N12_V9/Subsystem2 ==
  state : Inport
  vx : Inport  Port=2
  vy : Inport  Port=3
  vz : Inport  Port=4
  yaw : Inport  Port=5
  Enable : EnablePort
  Blank Message : robotlib/Blank Message  messageClass=Message  entityType=std_msgs/UInt64  messageType=std_msgs/UInt64  SampleTime=inf
  Blank Message1 : robotlib/Blank Message  messageClass=Message  entityType=geometry_msgs/TwistStamped  messageType=geometry_msgs/TwistStamped  SampleTime=inf
  Bus Assignment : BusAssignment  AssignedSignals=Data
  Bus Assignment1 : BusAssignment  AssignedSignals=Twist.Linear.X,Twist.Linear.Y,Twist.Linear.Z,Twist.Angular.Z
  Publish : robotlib/Publish  topicSource=Select from ROS network  topic=/drone_3/state  messageType=std_msgs/UInt64  messageQueueLength=1
  Publish1 : robotlib/Publish  topicSource=Select from ROS network  topic=/drone_3/mavros/setpoint_velocity/cmd_vel  messageType=geometry_msgs/TwistStamped  messageQueueLength=1
  wires:
  Blank Message/1 -> Bus Assignment/1
  state/1 -> Bus Assignment/2
  Bus Assignment/1 -> Publish/1
  Bus Assignment1/1 -> Publish1/1
  Blank Message1/1 -> Bus Assignment1/1
  vx/1 -> Bus Assignment1/2
  vy/1 -> Bus Assignment1/3
  yaw/1 -> Bus Assignment1/5
  vz/1 -> Bus Assignment1/4

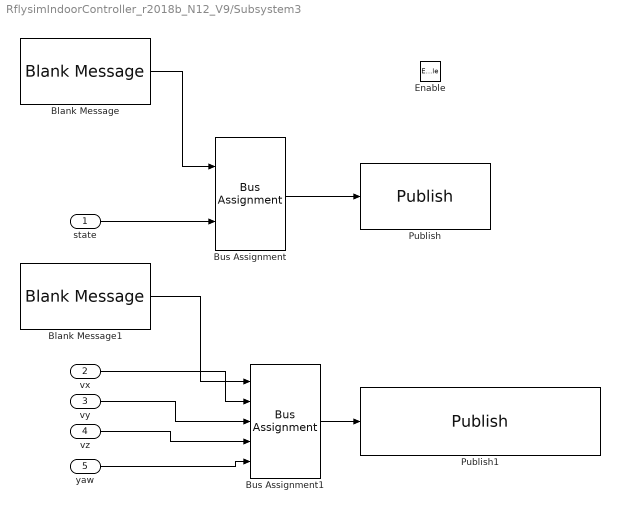
== system RflysimIndoorController_r2018b_N12_V9/Subsystem3 ==
  state : Inport
  vx : Inport  Port=2
  vy : Inport  Port=3
  vz : Inport  Port=4
  yaw : Inport  Port=5
  Enable : EnablePort
  Blank Message : robotlib/Blank Message  messageClass=Message  entityType=std_msgs/UInt64  messageType=std_msgs/UInt64  SampleTime=inf
  Blank Message1 : robotlib/Blank Message  messageClass=Message  entityType=geometry_msgs/TwistStamped  messageType=geometry_msgs/TwistStamped  SampleTime=inf
  Bus Assignment : BusAssignment  AssignedSignals=Data
  Bus Assignment1 : BusAssignment  AssignedSignals=Twist.Linear.X,Twist.Linear.Y,Twist.Linear.Z,Twist.Angular.Z
  Publish : robotlib/Publish  topicSource=Specify your own  topic=/drone_4/state  messageType=std_msgs/UInt64  messageQueueLength=1
  Publish1 : robotlib/Publish  topicSource=Specify your own  topic=/drone_4/mavros/setpoint_velocity/cmd_vel  messageType=geometry_msgs/TwistStamped  messageQueueLength=1
  wires:
  Blank Message/1 -> Bus Assignment/1
  state/1 -> Bus Assignment/2
  Bus Assignment/1 -> Publish/1
  Bus Assignment1/1 -> Publish1/1
  Blank Message1/1 -> Bus Assignment1/1
  vx/1 -> Bus Assignment1/2
  vy/1 -> Bus Assignment1/3
  yaw/1 -> Bus Assignment1/5
  vz/1 -> Bus Assignment1/4

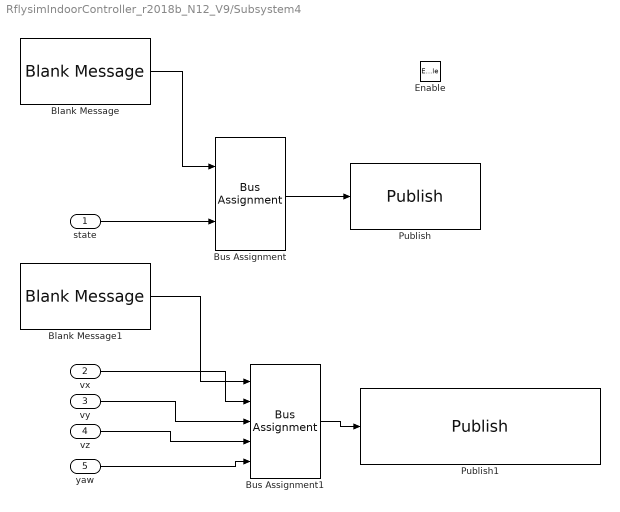
== system RflysimIndoorController_r2018b_N12_V9/Subsystem4 ==
  state : Inport
  vx : Inport  Port=2
  vy : Inport  Port=3
  vz : Inport  Port=4
  yaw : Inport  Port=5
  Enable : EnablePort
  Blank Message : robotlib/Blank Message  messageClass=Message  entityType=std_msgs/UInt64  messageType=std_msgs/UInt64  SampleTime=inf
  Blank Message1 : robotlib/Blank Message  messageClass=Message  entityType=geometry_msgs/TwistStamped  messageType=geometry_msgs/TwistStamped  SampleTime=inf
  Bus Assignment : BusAssignment  AssignedSignals=Data
  Bus Assignment1 : BusAssignment  AssignedSignals=Twist.Linear.X,Twist.Linear.Y,Twist.Linear.Z,Twist.Angular.Z
  Publish : robotlib/Publish  topicSource=Specify your own  topic=/drone_5/state  messageType=std_msgs/UInt64  messageQueueLength=1
  Publish1 : robotlib/Publish  topicSource=Specify your own  topic=/drone_5/mavros/setpoint_velocity/cmd_vel  messageType=geometry_msgs/TwistStamped  messageQueueLength=1
  wires:
  Blank Message/1 -> Bus Assignment/1
  state/1 -> Bus Assignment/2
  Bus Assignment/1 -> Publish/1
  Bus Assignment1/1 -> Publish1/1
  Blank Message1/1 -> Bus Assignment1/1
  vx/1 -> Bus Assignment1/2
  vy/1 -> Bus Assignment1/3
  yaw/1 -> Bus Assignment1/5
  vz/1 -> Bus Assignment1/4

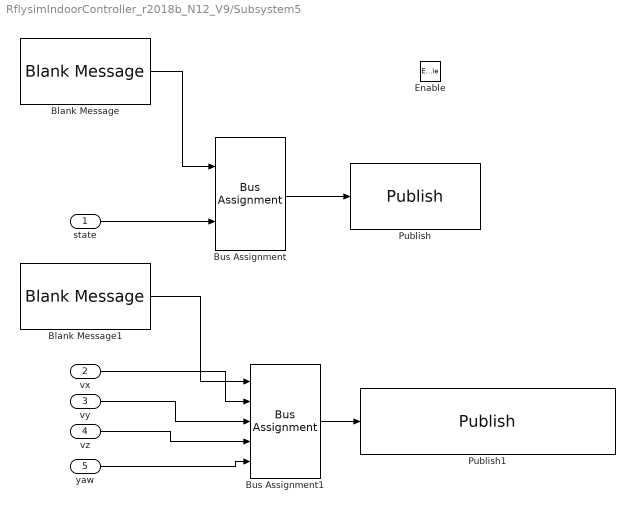
== system RflysimIndoorController_r2018b_N12_V9/Subsystem5 ==
  state : Inport
  vx : Inport  Port=2
  vy : Inport  Port=3
  vz : Inport  Port=4
  yaw : Inport  Port=5
  Enable : EnablePort
  Blank Message : robotlib/Blank Message  messageClass=Message  entityType=std_msgs/UInt64  messageType=std_msgs/UInt64  SampleTime=inf
  Blank Message1 : robotlib/Blank Message  messageClass=Message  entityType=geometry_msgs/TwistStamped  messageType=geometry_msgs/TwistStamped  SampleTime=inf
  Bus Assignment : BusAssignment  AssignedSignals=Data
  Bus Assignment1 : BusAssignment  AssignedSignals=Twist.Linear.X,Twist.Linear.Y,Twist.Linear.Z,Twist.Angular.Z
  Publish : robotlib/Publish  topicSource=Specify your own  topic=/drone_6/state  messageType=std_msgs/UInt64  messageQueueLength=1
  Publish1 : robotlib/Publish  topicSource=Specify your own  topic=/drone_6/mavros/setpoint_velocity/cmd_vel  messageType=geometry_msgs/TwistStamped  messageQueueLength=1
  wires:
  Blank Message/1 -> Bus Assignment/1
  state/1 -> Bus Assignment/2
  Bus Assignment/1 -> Publish/1
  Bus Assignment1/1 -> Publish1/1
  Blank Message1/1 -> Bus Assignment1/1
  vx/1 -> Bus Assignment1/2
  vy/1 -> Bus Assignment1/3
  yaw/1 -> Bus Assignment1/5
  vz/1 -> Bus Assignment1/4

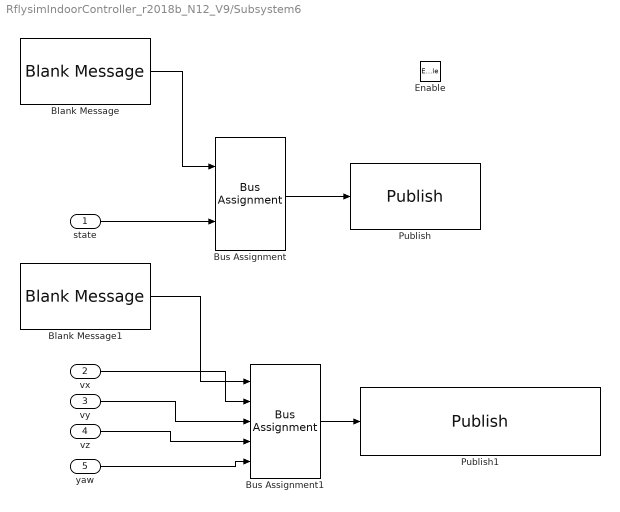
== system RflysimIndoorController_r2018b_N12_V9/Subsystem6 ==
  state : Inport
  vx : Inport  Port=2
  vy : Inport  Port=3
  vz : Inport  Port=4
  yaw : Inport  Port=5
  Enable : EnablePort
  Blank Message : robotlib/Blank Message  messageClass=Message  entityType=std_msgs/UInt64  messageType=std_msgs/UInt64  SampleTime=inf
  Blank Message1 : robotlib/Blank Message  messageClass=Message  entityType=geometry_msgs/TwistStamped  messageType=geometry_msgs/TwistStamped  SampleTime=inf
  Bus Assignment : BusAssignment  AssignedSignals=Data
  Bus Assignment1 : BusAssignment  AssignedSignals=Twist.Linear.X,Twist.Linear.Y,Twist.Linear.Z,Twist.Angular.Z
  Publish : robotlib/Publish  topicSource=Specify your own  topic=/drone_7/state  messageType=std_msgs/UInt64  messageQueueLength=1
  Publish1 : robotlib/Publish  topicSource=Specify your own  topic=/drone_7/mavros/setpoint_velocity/cmd_vel  messageType=geometry_msgs/TwistStamped  messageQueueLength=1
  wires:
  Blank Message/1 -> Bus Assignment/1
  state/1 -> Bus Assignment/2
  Bus Assignment/1 -> Publish/1
  Bus Assignment1/1 -> Publish1/1
  Blank Message1/1 -> Bus Assignment1/1
  vx/1 -> Bus Assignment1/2
  vy/1 -> Bus Assignment1/3
  yaw/1 -> Bus Assignment1/5
  vz/1 -> Bus Assignment1/4

== system RflysimIndoorController_r2018b_N12_V9/Subsystem7 ==
  state : Inport
  vx : Inport  Port=2
  vy : Inport  Port=3
  vz : Inport  Port=4
  yaw : Inport  Port=5
  Enable : EnablePort
  Blank Message : robotlib/Blank Message  messageClass=Message  entityType=std_msgs/UInt64  messageType=std_msgs/UInt64  SampleTime=inf
  Blank Message1 : robotlib/Blank Message  messageClass=Message  entityType=geometry_msgs/TwistStamped  messageType=geometry_msgs/TwistStamped  SampleTime=inf
  Bus Assignment : BusAssignment  AssignedSignals=Data
  Bus Assignment1 : BusAssignment  AssignedSignals=Twist.Linear.X,Twist.Linear.Y,Twist.Linear.Z,Twist.Angular.Z
  Publish : robotlib/Publish  topicSource=Specify your own  topic=/drone_8/state  messageType=std_msgs/UInt64  messageQueueLength=1
  Publish1 : robotlib/Publish  topicSource=Specify your own  topic=/drone_8/mavros/setpoint_velocity/cmd_vel  messageType=geometry_msgs/TwistStamped  messageQueueLength=1
  wires:
  Blank Message/1 -> Bus Assignment/1
  state/1 -> Bus Assignment/2
  Bus Assignment/1 -> Publish/1
  Bus Assignment1/1 -> Publish1/1
  Blank Message1/1 -> Bus Assignment1/1
  vx/1 -> Bus Assignment1/2
  vy/1 -> Bus Assignment1/3
  yaw/1 -> Bus Assignment1/5
  vz/1 -> Bus Assignment1/4

== system RflysimIndoorController_r2018b_N12_V9/Subsystem8 ==
  state : Inport
  vx : Inport  Port=2
  vy : Inport  Port=3
  vz : Inport  Port=4
  yaw : Inport  Port=5
  Enable : EnablePort
  Blank Message : robotlib/Blank Message  messageClass=Message  entityType=std_msgs/UInt64  messageType=std_msgs/UInt64  SampleTime=inf
  Blank Message1 : robotlib/Blank Message  messageClass=Message  entityType=geometry_msgs/TwistStamped  messageType=geometry_msgs/TwistStamped  SampleTime=inf
  Bus Assignment : BusAssignment  AssignedSignals=Data
  Bus Assignment1 : BusAssignment  AssignedSignals=Twist.Linear.X,Twist.Linear.Y,Twist.Linear.Z,Twist.Angular.Z
  Publish : robotlib/Publish  topicSource=Specify your own  topic=/drone_9/state  messageType=std_msgs/UInt64  messageQueueLength=1
  Publish1 : robotlib/Publish  topicSource=Specify your own  topic=/drone_9/mavros/setpoint_velocity/cmd_vel  messageType=geometry_msgs/TwistStamped  messageQueueLength=1
  wires:
  Blank Message/1 -> Bus Assignment/1
  state/1 -> Bus Assignment/2
  Bus Assignment/1 -> Publish/1
  Bus Assignment1/1 -> Publish1/1
  Blank Message1/1 -> Bus Assignment1/1
  vx/1 -> Bus Assignment1/2
  vy/1 -> Bus Assignment1/3
  yaw/1 -> Bus Assignment1/5
  vz/1 -> Bus Assignment1/4

== system RflysimIndoorController_r2018b_N12_V9/Subsystem9 ==
  state : Inport
  vx : Inport  Port=2
  vy : Inport  Port=3
  vz : Inport  Port=4
  yaw : Inport  Port=5
  Enable : EnablePort
  Blank Message : robotlib/Blank Message  messageClass=Message  entityType=std_msgs/UInt64  messageType=std_msgs/UInt64  SampleTime=inf
  Blank Message1 : robotlib/Blank Message  messageClass=Message  entityType=geometry_msgs/TwistStamped  messageType=geometry_msgs/TwistStamped  SampleTime=inf
  Bus Assignment : BusAssignment  AssignedSignals=Data
  Bus Assignment1 : BusAssignment  AssignedSignals=Twist.Linear.X,Twist.Linear.Y,Twist.Linear.Z,Twist.Angular.Z
  Publish : robotlib/Publish  topicSource=Specify your own  topic=/drone_10/state  messageType=std_msgs/UInt64  messageQueueLength=1
  Publish1 : robotlib/Publish  topicSource=Specify your own  topic=/drone_10/mavros/setpoint_velocity/cmd_vel  messageType=geometry_msgs/TwistStamped  messageQueueLength=1
  wires:
  Blank Message/1 -> Bus Assignment/1
  state/1 -> Bus Assignment/2
  Bus Assignment/1 -> Publish/1
  Bus Assignment1/1 -> Publish1/1
  Blank Message1/1 -> Bus Assignment1/1
  vx/1 -> Bus Assignment1/2
  vy/1 -> Bus Assignment1/3
  yaw/1 -> Bus Assignment1/5
  vz/1 -> Bus Assignment1/4

== matlab function RflysimIndoorController_r2018b_N12_V9/MATLAB Function1 ==
  data: states input; tunnel_msg1 input; tunnel_msg2 input; tunnel_msg3 input; ux output; uy output; p_target input; Pcur input; Vcur input; Yawcur input; gain input; vmax input; uyaw output; rs input; ra input; states_new output; p_radius output; p_left_encircle output; p_right_encircle output
function [ux,uy,uyaw,states_new,p_radius,p_left_encircle,p_right_encircle]  = mytunnel(states,tunnel_msg1,tunnel_msg2,tunnel_msg3,p_target,Pcur,Vcur,Yawcur,gain,vmax,rs,ra)
p_target=p_target';

N=3;
ux=zeros(N,1);
uy=zeros(N,1);
uyaw=zeros(N,1);
states_new=zeros(N,1);
tunnel_msg=tunnel_msg1;    
for j=1:N
    
    left_x=zeros(10,1);
    left_y=zeros(10,1);
    right_x=zeros(10,1);
    right_y=zeros(10,1);
    middle_x=zeros(10,1);
    middle_y=zeros(10,1);
    if j==1
        tunnel_msg=tunnel_msg1;
    elseif j==2
        tunnel_msg=tunnel_msg2;
    elseif j==3
        tunnel_msg=tunnel_msg3;
    end
    
    tunnel_type = tunnel_msg.Pipetype.Data;
    point_num=tunnel_msg.Units_SL_Info.CurrentLength;
    
    for k=1:point_num
        left_x(k,1) = tunnel_msg.Units(k).Left.X;
        left_y(k,1) = tunnel_msg.Units(k).Left.Y;
        
        right_x(k,1) = tunnel_msg.Units(k).Right.X;
        right_y(k,1) = tunnel_msg.Units(k).Right.Y;
        
        middle_x(k,1) = tunnel_msg.Units(k).Middle.X;
        middle_y(k,1) = tunnel_msg.Units(k).Middle.Y;
    end
    
    left_x=left_x(1:point_num,1);
    left_y=left_y(1:point_num,1);
    right_x=right_x(1:point_num,1);
    right_y=right_y(1:point_num,1);
    middle_x=middle_x(1:point_num,1);
    middle_y=middle_y(1:point_num,1);

    inter_num = 100;
    p_radius=zeros(inter_num,2);
    p_left_encircle=zeros(inter_num,2);
    p_right_encircle=zeros(inter_num,2);
    
    if tunnel_type==10
        k=1:length(middle_x);
        ki=linspace(1,length(middle_x),inter_num); %%%%% 插值的点越多，控制更精确，曲线更光滑，计算更耗时
        p_radius_x=(interp1(k,middle_x,ki,'pchip'))';
        p_radius_y=(interp1(k,middle_y,ki,'pchip'))';
        for i=1:length(p_radius(:,1))
            p_radius(i,1)=p_radius_x(i);
            p_radius(i,2)=p_radius_y(i);
        end
        
        k=1:length(left_x);
        ki=linspace(1,length(left_x),inter_num); %%%%% 插值的点越多，控制更精确，曲线更光滑，计算更耗时
        p_left_encircle_x=(interp1(k,left_x,ki,'pchip'))';
        p_left_encircle_y=(interp1(k,left_y,ki,'pchip'))';
        for i=1:length(p_left_encircle(:,1))
            p_left_encircle(i,1)=p_left_encircle_x(i);
            p_left_encircle(i,2)=p_left_encircle_y(i);
        end
        
        k=1:length(right_x);
        ki=linspace(1,length(right_x),inter_num); %%%%% 插值的点越多，控制更精确，曲线更光滑，计算更耗时
        p_right_encircle_x=(interp1(k,right_x,ki,'pchip'))';
        p_right_encircle_y=(interp1(k,right_y,ki,'pchip'))';
        for i=1:length(p_right_encircle(:,1))
            p_right_encircle(i,1)=p_right_encircle_x(i);
            p_right_encircle(i,2)=p_right_encircle_y(i);
        end
    end


    
    [u_encircle,ux_encircle,uy_encircle,uyaw_encircle,leader_locate,dist_encircle]  = Encirclement2(p_radius,p_left_encircle,p_right_encircle,p_target,Pcur,Vcur,Yawcur,gain,vmax,rs,ra,j);
    
    if states(j)==30
        states_new(j)=30;
        if tunnel_type==10
            ux(j)=ux_encircle;
            uy(j)=uy_encircle;
            uyaw(j)=uyaw_encircle;
            if abs(leader_locate-inter_num)<5
                states_new(j)=20;
            end
        end
    end
end
